simulink model "YAW_CONTROL_harness"  (R2020b)
settings: Solver=ode4  StartTime=0.0  StopTime=par.sym.Ttot  FixedStep=par.sym.max_dt  MaxStep=par.sym.max_dt  RelTol=1e-3
settings Model: Creator=carar  LastModifiedBy=carar
settings SolverCC: AlgebraicLoopSolver=LineSearch
settings DataIOCC: SaveOutput=off  SaveTime=off  ReturnWorkspaceOutputs=off  TimeSaveName=TIME
settings OptimizationCC: LifeSpan=inf
settings DebuggingCC: UnconnectedInputMsg=none  UnconnectedOutputMsg=none  ArithmeticOperatorsInVariantConditions=warning
settings SFSimCC: CustomCodeUndefinedFunction=UseInterfaceOnly
settings CodeAppCC: GenerateComments=off
settings SimscapeCC: SimscapeNormalizeSystem=off

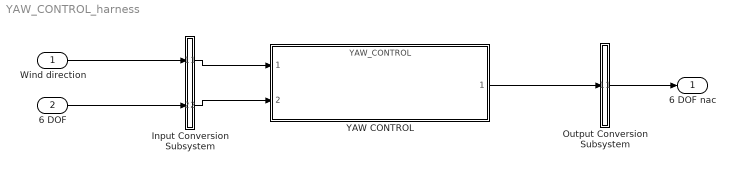
== system YAW_CONTROL_harness ==
  Wind direction : Inport  OutDataTypeStr=double  PortDimensions=[1]  SampleTime=0.05
  6 DOF : Inport  Port=2  OutDataTypeStr=double  PortDimensions=[18]  SampleTime=0.05
  Input Conversion Subsystem : Subsystem  Tag=__SLT_ICS__  Description=|
      | Signal spec.
      | and routing
      settings: AttributesFormatString=%<Description>
  Output Conversion Subsystem : Subsystem  Tag=__SLT_OCS__  Description=|
      | Signal spec.
      | and routing
      settings: AttributesFormatString=%<Description>
  YAW CONTROL : ModelReference  ModelNameDialog=YAW_CONTROL.slxp  ModelReferenceVersion=5.20  CopyOfModelProtected=on
  6 DOF nac : Outport
  wires:
  Wind direction/1 -> Input Conversion Subsystem/1(Inport_1)
  6 DOF/1 -> Input Conversion Subsystem/2(Inport_2)
  Output Conversion Subsystem/1(Outport_1) -> 6 DOF nac/1
  Input Conversion Subsystem/1(Outport_1) -> YAW CONTROL/1
  Input Conversion Subsystem/2(Outport_2) -> YAW CONTROL/2
  YAW CONTROL/1 -> Output Conversion Subsystem/1(Inport_1)

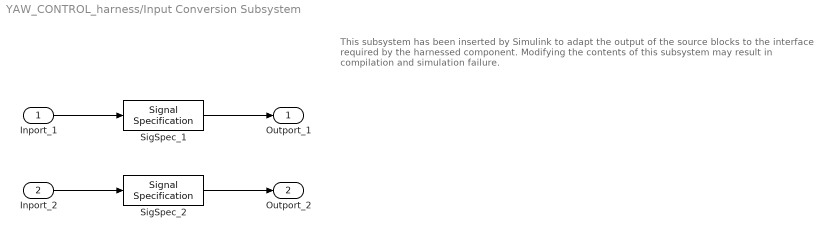
== system YAW_CONTROL_harness/Input Conversion Subsystem ==
  note: This subsystem has been inserted by Simulink to adapt the output of the source blocks to the interface required by the harnessed component.
      |  Modifying the contents of this subsystem may result in compilation and simulation failure.
  Inport_1 : Inport
  Inport_2 : Inport  Port=2
  SigSpec_1 : SignalSpecification  OutDataTypeStr=double  Dimensions=[1]  SampleTime=0.05
  SigSpec_2 : SignalSpecification  OutDataTypeStr=double  Dimensions=[18]  SampleTime=0.05
  Outport_1 : Outport
  Outport_2 : Outport  Port=2
  wires:
  SigSpec_1/1 -> Outport_1/1
  Inport_1/1 -> SigSpec_1/1
  SigSpec_2/1 -> Outport_2/1
  Inport_2/1 -> SigSpec_2/1

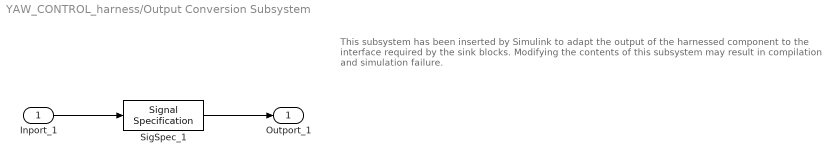
== system YAW_CONTROL_harness/Output Conversion Subsystem ==
  note: This subsystem has been inserted by Simulink to adapt the output of the harnessed component to the interface required by the sink blocks.
      |  Modifying the contents of this subsystem may result in compilation and simulation failure.
  Inport_1 : Inport
  SigSpec_1 : SignalSpecification  OutDataTypeStr=double  Dimensions=[18]  SampleTime=0.05
  Outport_1 : Outport
  wires:
  Inport_1/1 -> SigSpec_1/1
  SigSpec_1/1 -> Outport_1/1
